simulink model "IfElse"  (R2017b)
settings: Solver=FixedStepDiscrete  StartTime=0.0  StopTime=10.0  RelTol=1e-3
settings Model: Creator=engdo  LastModifiedBy=engdo
settings OptimizationCC: DefaultParameterBehavior=Inlined  PassReuseOutputArgsAs=Individual arguments
settings DebuggingCC: ParameterTunabilityLossMsg=error
settings SFSimCC: MATLABDynamicMemAlloc=off
settings RTWCC: SystemTargetFile=ert.tlc  GenCodeOnly=on  TemplateMakefile=ert_default_tmf  GenerateReport=on  IncludeHyperlinkInReport=on  LaunchReport=on  GenerateTraceInfo=on  GenerateTraceReport=on  GenerateTraceReportSl=on  GenerateTraceReportSf=on  GenerateTraceReportEml=on  GenerateWebview=on
settings CodeAppCC: ForceParamTrailComments=on  IgnoreCustomStorageClasses=off  OperatorAnnotations=on  SimulinkDataObjDesc=on  SFDataObjDesc=on  InsertBlockDesc=on
settings ERTTargetCC: TargetLangStandard=C99 (ISO)  GenerateSampleERTMain=on  InlinedParameterPlacement=NonHierarchical  ERTCustomFileTemplate=example_file_process.tlc  EnableUserReplacementTypes=on

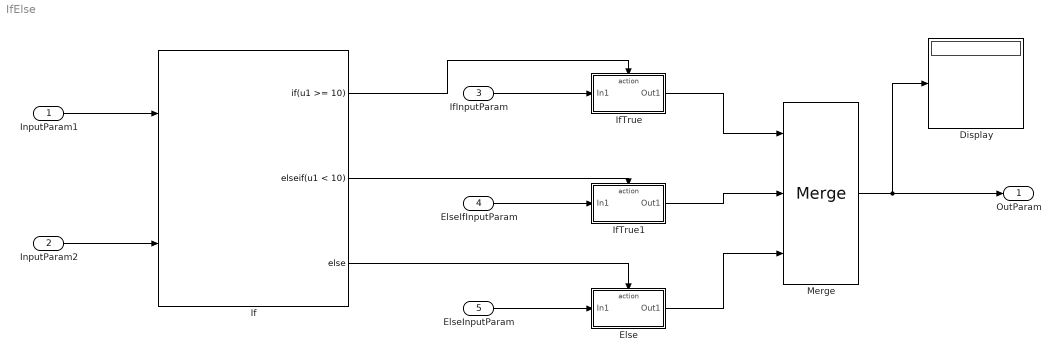
== system IfElse ==
  InputParam1 : Inport
  InputParam2 : Inport  Port=2
  IfInputParam : Inport  Port=3
  ElseIfInputParam : Inport  Port=4
  ElseInputParam : Inport  Port=5
  Display : Display
  Else : Subsystem  TreatAsAtomicUnit=on
  If : If  NumInputs=2  IfExpression=u1 >= 10  ElseIfExpressions=u1 < 10
  IfTrue : Subsystem  TreatAsAtomicUnit=on
  IfTrue1 : Subsystem  TreatAsAtomicUnit=on
  Merge : Merge  Inputs=3
  OutParam : Outport
  wires:
  If/3 -> Else/Action
  If/1 -> IfTrue/Action
  IfTrue/1(Out1) -> Merge/1
  Else/1(Out1) -> Merge/3
  Merge/1 -> Display/1, OutParam/1
  IfInputParam/1 -> IfTrue/1(In1)
  ElseInputParam/1 -> Else/1(In1)
  InputParam1/1 -> If/1
  InputParam2/1 -> If/2
  If/2 -> IfTrue1/Action
  ElseIfInputParam/1 -> IfTrue1/1(In1)
  IfTrue1/1(Out1) -> Merge/2

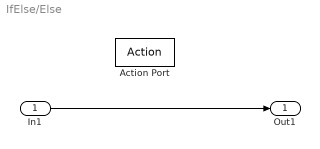
== system IfElse/Else ==
  In1 : Inport
  Action Port : ActionPort  ActionType=else
  Out1 : Outport
  wires:
  In1/1 -> Out1/1

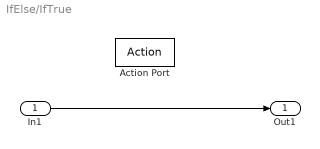
== system IfElse/IfTrue ==
  In1 : Inport
  Action Port : ActionPort  ActionType=then
  Out1 : Outport
  wires:
  In1/1 -> Out1/1

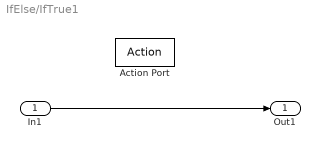
== system IfElse/IfTrue1 ==
  In1 : Inport
  Action Port : ActionPort  ActionType=elseif
  Out1 : Outport
  wires:
  In1/1 -> Out1/1
